simulink model "crop_simulation"  (R2021a)
settings: Solver=ode23tb  StartTime=0.0  StopTime=4  RelTol=1e-2
values from neighbouring files (symbols this model uses):
  parameters = LoadParameters()    [OnlyPlots.m]    (also in run_crop_simulation.m; run_several_crop_simulation.m)
undefined symbols (not defined in the file or in its folder): climate_GH3, MM_vec, nearst_p, p, PowerArtificial, Tr, Tref, Ts, x0_SOFC
libraries: HORTISIM x14, pid_lib x4
(part 3 of 3)

== system crop_simulation/Control Systems/Heater/SOFC cascada/Reformer + SOFC/Reformer  - SOFC System/SOFC /Nernst’s Eq  ==
  note: Hemos fijado la dimension de salida de este bloque
  note: 'H2' , 'O2' , 'H2O' , 'N2' , 'CO' , 'CH4' , 'CO2' , 'Diesel' ,'Ar','Csoot'
  Xa : Inport
  I : Inport  Port=2
  T : Inport  Port=3
  ratio a/c : Inport  Port=4
  Constant5 : Constant  Value=nearst_p.mu_out
  Gain : Gain  Gain=nearst_p.std_out
  MATLAB Function1 : MATLAB Function  TreatAsAtomicUnit=on
  Scope1 : Scope
  Subsystem : Subsystem
  Subsystem1 : Subsystem  Variant=on  VariantControlMode=label  VariantControl=Choice  LabelModeActiveChoice=Choice_1
  Sum : Sum  Inputs=|++
  V : Outport  PortDimensions=1
  wires:
  T/1 -> Subsystem/2(T)
  Xa/1 -> Subsystem/3(la)
  ratio a/c/1 -> Subsystem/1(ratio a/c)
  Gain/1 -> Sum/1
  Constant5/1 -> Sum/2
  Sum/1 -> Scope1/1, MATLAB Function1/1(params)
  MATLAB Function1/1(V) -> V/1
  I/1 -> MATLAB Function1/2(I)
  Subsystem/1(Out7) -> Subsystem1/1(In1)
  Subsystem1/1(Out1) -> Gain/1

== system crop_simulation/Control Systems/Heater/SOFC cascada/Reformer + SOFC/Reformer  - SOFC System/SOFC /Subsystem ==
  Air[mol/s] : Inport
  Molar Fractions (H2,O2,H2O,N2,CO,CH4,CO2) [mol/(Air-mol)] : Constant  Value=[0 0.2095 0 0.7808 0 0 0 0 0 0]
  Product : Product
  Cathode [mol/s] : Outport
  wires:
  Air[mol/s]/1 -> Product/1  "Air [mol/s]"
  Product/1 -> Cathode [mol/s]/1  "Cathode [mol/s]"
  Molar Fractions (H2,O2,H2O,N2,CO,CH4,CO2) [mol/(Air-mol)]/1 -> Product/2

== system crop_simulation/Control Systems/Heater/SOFC/Reformer  - SOFC System/Reformer /Subsystem/Subsystem/Subsystem ==
  In1 : Inport
  Equilibrium : MATLABFcn  MATLABFcn=forward_reformer_net  OutputDimensions=8  OutputSignalType=real  Output1D=off
  Out1 : Outport
  wires:
  In1/1 -> Equilibrium/1
  Equilibrium/1 -> Out1/1

== system crop_simulation/Control Systems/Heater/SOFC/Reformer  - SOFC System/Reformer /Subsystem/Subsystem/Subsystem1 ==
  In1 : Inport
  MATLAB Function : MATLAB Function  TreatAsAtomicUnit=on
  Out1 : Outport

== system crop_simulation/Control Systems/Heater/SOFC/Reformer  - SOFC System/Reformer /Subsystem/Subsystem1/Subsystem ==
  In1 : Inport
  MATLAB Function : MATLAB Function  TreatAsAtomicUnit=on
  Out1 : Outport

== system crop_simulation/Control Systems/Heater/SOFC/Reformer  - SOFC System/Reformer /Subsystem/Subsystem1/Subsystem1 ==
  In1 : Inport
  Inlet Composition : MATLABFcn  MATLABFcn=inlet_reformer_net  OutputDimensions=6  OutputSignalType=real  Output1D=off
  Out1 : Outport
  wires:
  In1/1 -> Inlet Composition/1
  Inlet Composition/1 -> Out1/1

== system crop_simulation/Control Systems/Heater/SOFC/Reformer  - SOFC System/SOFC /Nernst’s Eq /Subsystem1/Subsystem ==
  In1 : Inport
  MATLAB Function : MATLAB Function  TreatAsAtomicUnit=on
  Out1 : Outport
  wires:
  In1/1 -> MATLAB Function/1(u)
  MATLAB Function/1(y) -> Out1/1

== system crop_simulation/Control Systems/Heater/SOFC/Reformer  - SOFC System/SOFC /Nernst’s Eq /Subsystem1/Subsystem1 ==
  In1 : Inport
  Interpreted MATLAB Function : MATLABFcn  MATLABFcn=nearst_nn
  Out1 : Outport
  wires:
  In1/1 -> Interpreted MATLAB Function/1
  Interpreted MATLAB Function/1 -> Out1/1

== system crop_simulation/Control Systems/Heater/SOFC cascada/Control Operations Points/Control OP/Select Operation Point/Select Operation Point/If Action Subsystem ==
  Action Port : ActionPort
  Constant : Constant  Value=4
  Out1 : Outport
  wires:
  Constant/1 -> Out1/1

== system crop_simulation/Control Systems/Heater/SOFC cascada/Control Operations Points/Control OP/Select Operation Point/Select Operation Point/If Action Subsystem1 ==
  Action Port : ActionPort
  Constant : Constant  Value=3
  Out1 : Outport
  wires:
  Constant/1 -> Out1/1

== system crop_simulation/Control Systems/Heater/SOFC cascada/Control Operations Points/Control OP/Select Operation Point/Select Operation Point/If Action Subsystem2 ==
  Action Port : ActionPort
  Constant : Constant
  Out1 : Outport
  wires:
  Constant/1 -> Out1/1

== system crop_simulation/Control Systems/Heater/SOFC cascada/Control Operations Points/Control OP/Transformacion Flujos/If Action Subsystem/Subsystem ==
  Constant : Constant  Value=11.64
  Constant1 : Constant  Value=14.14
  Constant2 : Constant  Value=36.18
  Constant3 : Constant  Value=144
  Out Bus Element : Outport  PortName=OP  Element=Diesel [ml/min]
  Out Bus Element1 : Outport  PortName=OP  Element=Steam [ml/min]
  Out Bus Element2 : Outport  PortName=OP  Element=Air [NL/min]
  Out Bus Element3 : Outport  PortName=OP  Element=Air_cath [NL/min]
  wires:
  Constant1/1 -> Out Bus Element1/1
  Constant2/1 -> Out Bus Element2/1
  Constant/1 -> Out Bus Element/1
  Constant3/1 -> Out Bus Element3/1

== system crop_simulation/Control Systems/Heater/SOFC cascada/Control Operations Points/Control OP/Transformacion Flujos/If Action Subsystem1/Subsystem1 ==
  Constant : Constant  Value=7.83
  Constant1 : Constant  Value=9.51
  Constant2 : Constant  Value=24.34
  Constant3 : Constant  Value=96
  Out Bus Element : Outport  PortName=OP  Element=Diesel [ml/min]
  Out Bus Element1 : Outport  PortName=OP  Element=Steam [ml/min]
  Out Bus Element2 : Outport  PortName=OP  Element=Air [NL/min]
  Out Bus Element3 : Outport  PortName=OP  Element=Air_cath [NL/min]
  wires:
  Constant1/1 -> Out Bus Element1/1
  Constant2/1 -> Out Bus Element2/1
  Constant/1 -> Out Bus Element/1
  Constant3/1 -> Out Bus Element3/1

== system crop_simulation/Control Systems/Heater/SOFC cascada/Control Operations Points/Control OP/Transformacion Flujos/If Action Subsystem2/Subsystem2 ==
  Constant : Constant  Value=6.51
  Constant1 : Constant  Value=7.91
  Constant2 : Constant  Value=20.24
  Constant3 : Constant  Value=80
  Out Bus Element : Outport  PortName=OP  Element=Diesel [ml/min]
  Out Bus Element1 : Outport  PortName=OP  Element=Steam [ml/min]
  Out Bus Element2 : Outport  PortName=OP  Element=Air [NL/min]
  Out Bus Element3 : Outport  PortName=OP  Element=Air_cath [NL/min]
  wires:
  Constant1/1 -> Out Bus Element1/1
  Constant2/1 -> Out Bus Element2/1
  Constant/1 -> Out Bus Element/1
  Constant3/1 -> Out Bus Element3/1

== system crop_simulation/Control Systems/Heater/SOFC cascada/Control Operations Points/Control OP/Transformacion Flujos/If Action Subsystem3/Subsystem2 ==
  Constant : Constant  Value=4.41
  Constant1 : Constant  Value=5.36
  Constant2 : Constant  Value=13.72
  Constant3 : Constant  Value=55
  Out Bus Element : Outport  PortName=OP  Element=Diesel [ml/min]
  Out Bus Element1 : Outport  PortName=OP  Element=Steam [ml/min]
  Out Bus Element2 : Outport  PortName=OP  Element=Air [NL/min]
  Out Bus Element3 : Outport  PortName=OP  Element=Air_cath [NL/min]
  wires:
  Constant1/1 -> Out Bus Element1/1
  Constant2/1 -> Out Bus Element2/1
  Constant/1 -> Out Bus Element/1
  Constant3/1 -> Out Bus Element3/1

== system crop_simulation/Control Systems/Heater/SOFC cascada/Reformer + SOFC/Reformer  - SOFC System/Reformer /Subsystem/Order Data ==
  note: Target
  note: Target
  note: 'H2' , 'O2' , 'H2O' , 'N2' , 'CO' , 'CH4' , 'CO2' , 'Diesel' ,'Ar','Csoot'
  In1 : Inport
  Demux : Demux  Outputs=8
  Vector Concatenate : Concatenate  NumInputs=10
  Out1 : Outport
  wires:
  In1/1 -> Demux/1
  Demux/1 -> [Ar]
  Demux/2 -> [CH4]
  Demux/3 -> [CO]
  Demux/4 -> [CO2]
  Demux/5 -> [H2]
  Demux/6 -> [H2O]
  Demux/7 -> [N2]
  Demux/8 -> [Csoot]
  [H2] -> Vector Concatenate/1
  [H2O] -> Vector Concatenate/3
  [N2] -> Vector Concatenate/4
  [CO] -> Vector Concatenate/5
  [CH4] -> Vector Concatenate/6
  [CO2] -> Vector Concatenate/7
  [Ar] -> Vector Concatenate/9
  [Csoot] -> Vector Concatenate/10
  Vector Concatenate/1 -> Out1/1

== system crop_simulation/Control Systems/Heater/SOFC cascada/Reformer + SOFC/Reformer  - SOFC System/Reformer /Subsystem/Order Data1 ==
  note: 'H2' , 'O2' , 'H2O' , 'N2' , 'CO' , 'CH4' , 'CO2' , 'Diesel' ,'Ar','Csoot'
  In1 : Inport
  Demux : Demux  Outputs=6
  Vector Concatenate : Concatenate  NumInputs=10
  Out1 : Outport
  wires:
  In1/1 -> Demux/1
  Demux/1 -> [N2]
  Demux/2 -> [O2]
  Demux/3 -> [CO2]
  Demux/4 -> [H2O]
  Demux/5 -> [Ar]
  Demux/6 -> [Diesel]
  [H2O] -> Vector Concatenate/3
  [N2] -> Vector Concatenate/4
  [CO2] -> Vector Concatenate/7
  [Ar] -> Vector Concatenate/9
  Vector Concatenate/1 -> Out1/1
  [O2] -> Vector Concatenate/2
  [Diesel] -> Vector Concatenate/8

== system crop_simulation/Control Systems/Heater/SOFC cascada/Reformer + SOFC/Reformer  - SOFC System/Reformer /Subsystem/Subsystem ==
  In1 : Inport
  Subsystem : Subsystem  VariantControl=Choice
  Subsystem1 : Subsystem  VariantControl=Choice_1
  Out1 : Outport

== system crop_simulation/Control Systems/Heater/SOFC cascada/Reformer + SOFC/Reformer  - SOFC System/Reformer /Subsystem/Subsystem1 ==
  In1 : Inport
  Subsystem : Subsystem  VariantControl=Choice_1
  Subsystem1 : Subsystem  VariantControl=Choice
  Out1 : Outport

== system crop_simulation/Control Systems/Heater/SOFC cascada/Reformer + SOFC/Reformer  - SOFC System/Reformer /Subsystem1/Ainhoa ==
  Mass Flow : Inport
  T : Inport  Port=2
  Deactivation : Subsystem  mask{k0=parameters.Heating.Reformer.deactivation.k0, k=parameters.Heating.Reformer.deactivation.k, nd=parameters.Heating.Reformer.deactivation.nd, Kw_ast=parameters.Heating.Reformer.deactivation.Kw_ast, Ew=parameters.Heating.Reformer.deactivation.Ew}
  activity : Outport
  wires:
  Deactivation/1(Out1) -> activity/1
  Mass Flow/1 -> Deactivation/1(mf)
  T/1 -> Deactivation/2(T)

== system crop_simulation/Control Systems/Heater/SOFC cascada/Reformer + SOFC/Reformer  - SOFC System/Reformer /Subsystem1/Simple ==
  Gain : Gain  Gain=0
  Integrator : Integrator  InitialCondition=1
  seconds 2 days1 : Gain  Gain=3600*24*0.001
  activity : Outport
  wires:
  Integrator/1 -> activity/1, Gain/1
  seconds 2 days1/1 -> Integrator/1
  Gain/1 -> seconds 2 days1/1

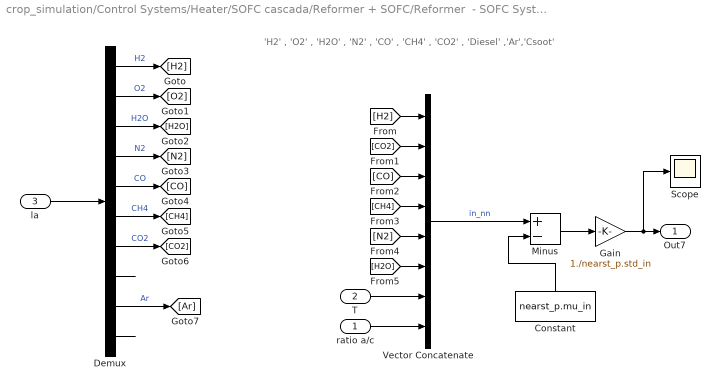
== system crop_simulation/Control Systems/Heater/SOFC cascada/Reformer + SOFC/Reformer  - SOFC System/SOFC /Nernst’s Eq /Subsystem ==
  note: 'H2' , 'O2' , 'H2O' , 'N2' , 'CO' , 'CH4' , 'CO2' , 'Diesel' ,'Ar','Csoot'
  ratio a/c : Inport
  T : Inport  Port=2
  la : Inport  Port=3
  Constant : Constant  Value=nearst_p.mu_in
  Demux : Demux  Outputs=10
  Gain : Gain  Gain=1./nearst_p.std_in
  Minus : Sum  Inputs=+-
  Scope : Scope
  Vector Concatenate : Concatenate  NumInputs=8
  Out7 : Outport
  wires:
  Demux/7 -> [CO2]  "CO2"
  la/1 -> Demux/1
  Demux/3 -> [H2O]  "H2O"
  Demux/1 -> [H2]  "H2"
  Demux/8 -> ?
  Demux/2 -> [O2]  "O2"
  Demux/10 -> ?
  Demux/9 -> [Ar]  "Ar"
  Demux/5 -> [CO]  "CO"
  Demux/4 -> [N2]  "N2"
  Demux/6 -> [CH4]  "CH4"
  ratio a/c/1 -> Vector Concatenate/8
  T/1 -> Vector Concatenate/7
  [H2] -> Vector Concatenate/1
  [CO2] -> Vector Concatenate/2
  [CO] -> Vector Concatenate/3
  [CH4] -> Vector Concatenate/4
  [N2] -> Vector Concatenate/5
  [H2O] -> Vector Concatenate/6
  Vector Concatenate/1 -> Minus/1  "in_nn"
  Constant/1 -> Minus/2
  Minus/1 -> Gain/1
  Gain/1 -> Scope/1, Out7/1

== system crop_simulation/Control Systems/Heater/SOFC cascada/Reformer + SOFC/Reformer  - SOFC System/SOFC /Nernst’s Eq /Subsystem1 ==
  In1 : Inport
  Subsystem : Subsystem  VariantControl=Choice_1
  Subsystem1 : Subsystem  VariantControl=Choice
  Out1 : Outport

== system crop_simulation/Control Systems/Heater/SOFC cascada/Reformer + SOFC/Reformer  - SOFC System/Reformer /Subsystem/Subsystem/Subsystem ==
  In1 : Inport
  Equilibrium : MATLABFcn  MATLABFcn=forward_reformer_net  OutputDimensions=8  OutputSignalType=real  Output1D=off
  Out1 : Outport
  wires:
  In1/1 -> Equilibrium/1
  Equilibrium/1 -> Out1/1

== system crop_simulation/Control Systems/Heater/SOFC cascada/Reformer + SOFC/Reformer  - SOFC System/Reformer /Subsystem/Subsystem/Subsystem1 ==
  In1 : Inport
  MATLAB Function : MATLAB Function  TreatAsAtomicUnit=on
  Out1 : Outport
  wires:
  In1/1 -> MATLAB Function/1(u)
  MATLAB Function/1(y) -> Out1/1

== system crop_simulation/Control Systems/Heater/SOFC cascada/Reformer + SOFC/Reformer  - SOFC System/Reformer /Subsystem/Subsystem1/Subsystem ==
  In1 : Inport
  MATLAB Function : MATLAB Function  TreatAsAtomicUnit=on
  Out1 : Outport
  wires:
  In1/1 -> MATLAB Function/1(u)
  MATLAB Function/1(y) -> Out1/1

== system crop_simulation/Control Systems/Heater/SOFC cascada/Reformer + SOFC/Reformer  - SOFC System/Reformer /Subsystem/Subsystem1/Subsystem1 ==
  In1 : Inport
  Inlet Composition : MATLABFcn  MATLABFcn=inlet_reformer_net  OutputDimensions=6  OutputSignalType=real  Output1D=off
  Out1 : Outport
  wires:
  In1/1 -> Inlet Composition/1
  Inlet Composition/1 -> Out1/1

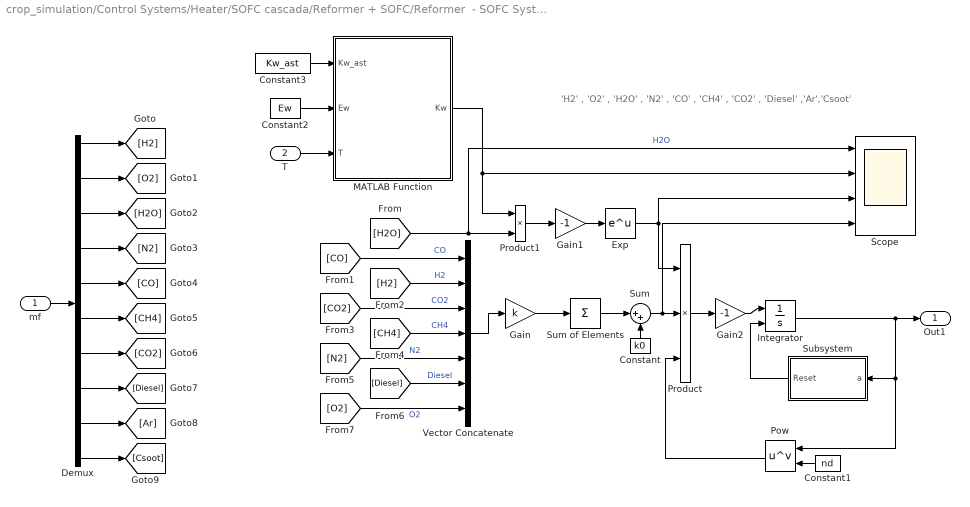
== system crop_simulation/Control Systems/Heater/SOFC cascada/Reformer + SOFC/Reformer  - SOFC System/Reformer /Subsystem1/Ainhoa/Deactivation ==
  note: 'H2' , 'O2' , 'H2O' , 'N2' , 'CO' , 'CH4' , 'CO2' , 'Diesel' ,'Ar','Csoot'
  mf : Inport
  T : Inport  Port=2
  Constant : Constant  Value=k0
  Constant1 : Constant  Value=nd
  Constant2 : Constant  Value=Ew
  Constant3 : Constant  Value=Kw_ast
  Demux : Demux  Outputs=10
  Exp : Math  SaturateOnIntegerOverflow=on
  Gain : Gain  Gain=k
  Gain1 : Gain  Gain=-1
  Gain2 : Gain  Gain=-1
  Integrator : Integrator  ExternalReset=rising  InitialCondition=1
  MATLAB Function : MATLAB Function  TreatAsAtomicUnit=on
  Pow : Math  Operator=pow  RndMeth=Zero  SaturateOnIntegerOverflow=on
  Product : Product  Inputs=3
  Product1 : Product
  Scope : Scope  NumInputPorts=4
  Subsystem : Subsystem
  Sum : Sum  Inputs=|++
  Sum of Elements : Sum  Inputs=+
  Vector Concatenate : Concatenate  NumInputs=7
  Out1 : Outport
  wires:
  Integrator/1 -> Out1/1, Subsystem/1(a), Pow/1
  mf/1 -> Demux/1
  [N2] -> Vector Concatenate/5  "N2"
  [CH4] -> Vector Concatenate/4  "CH4"
  [CO2] -> Vector Concatenate/3  "CO2"
  [H2] -> Vector Concatenate/2  "H2"
  [CO] -> Vector Concatenate/1  "CO"
  Vector Concatenate/1 -> Gain/1
  Constant/1 -> Sum/2
  Sum/1 -> Scope/4, Product/2
  [H2O] -> Scope/1, Product1/2  "H2O"
  Exp/1 -> Product/1, Scope/3
  Pow/1 -> Product/3
  Constant1/1 -> Pow/2
  Gain/1 -> Sum of Elements/1
  Sum of Elements/1 -> Sum/1
  Product/1 -> Gain2/1
  Gain2/1 -> Integrator/1
  [Diesel] -> Vector Concatenate/6  "Diesel"
  T/1 -> MATLAB Function/3(T)
  Constant2/1 -> MATLAB Function/2(Ew)
  Constant3/1 -> MATLAB Function/1(Kw_ast)
  MATLAB Function/1(Kw) -> Product1/1, Scope/2
  Product1/1 -> Gain1/1
  Gain1/1 -> Exp/1
  [O2] -> Vector Concatenate/7  "O2"
  Demux/1 -> [H2]
  Demux/2 -> [O2]
  Demux/3 -> [H2O]
  Demux/4 -> [N2]
  Demux/5 -> [CO]
  Demux/6 -> [CH4]
  Demux/7 -> [CO2]
  Demux/8 -> [Diesel]
  Demux/9 -> [Ar]
  Demux/10 -> [Csoot]
  Subsystem/1(Reset) -> Integrator/2

== system crop_simulation/Control Systems/Heater/SOFC cascada/Reformer + SOFC/Reformer  - SOFC System/SOFC /Nernst’s Eq /Subsystem1/Subsystem ==
  In1 : Inport
  MATLAB Function : MATLAB Function  TreatAsAtomicUnit=on
  Out1 : Outport
  wires:
  In1/1 -> MATLAB Function/1(u)
  MATLAB Function/1(y) -> Out1/1

== system crop_simulation/Control Systems/Heater/SOFC cascada/Reformer + SOFC/Reformer  - SOFC System/SOFC /Nernst’s Eq /Subsystem1/Subsystem1 ==
  In1 : Inport
  Interpreted MATLAB Function : MATLABFcn  MATLABFcn=nearst_nn
  Out1 : Outport
  wires:
  In1/1 -> Interpreted MATLAB Function/1
  Interpreted MATLAB Function/1 -> Out1/1

== system crop_simulation/Control Systems/Heater/SOFC cascada/Reformer + SOFC/Reformer  - SOFC System/Reformer /Subsystem1/Ainhoa/Deactivation/Subsystem ==
  a : Inport
  Constant : Constant
  Constant1 : Constant  Value=parameters.Heating.Reformer.deactivation.activity_threshold
  Delay : Delay  DelayLength=1  SampleTime=0.5/24
  Minus : Sum  Inputs=+-
  Minus1 : Sum  Inputs=+-
  Scope : Scope  NumInputPorts=2
  Sign : Signum
  Reset : Outport
  wires:
  Sign/1 -> Minus1/2
  Constant1/1 -> Minus/2
  Minus/1 -> Sign/1
  Constant/1 -> Minus1/1
  Minus1/1 -> Scope/2, Reset/1
  a/1 -> Scope/1, Delay/1
  Delay/1 -> Minus/1

== matlab function crop_simulation/Control Systems/Heater/SOFC cascada/Reformer + SOFC/Reformer  - SOFC System/Reformer /Subsystem/Subsystem1/Subsystem/MATLAB Function ==
  data: u input; y output
function y = fcn(u)

y = inlet_reformer_net(u);

== matlab function crop_simulation/Control Systems/Heater/SOFC cascada/Reformer + SOFC/Reformer  - SOFC System/SOFC /Anode/MATLAB Function ==
  data: qa_in input; ra output; I input; la output; pc_O2 input; pa input
function [ra,la] = fcn(qa_in,I,pc_O2,pa)

la = qa_in/sum(qa_in);


l_H2  = la(1);
%l_O2  = l(2);
%l_H2O = l(3);
%l_N2  = l(4);
l_CO  = la(5);
l_CH4 = la(6);
%l_CO2 = l(7);
%
alpha_H2 = l_H2;
alpha_CO  = l_CO;
alpha_CH4 = l_CH4;
%alpha_O2  = 0.5*(l_H2+l_CO+4*l_CH4);
beta_H2O  = l_H2 + 2*l_CH4;
beta_CO2  = l_CO + l_CH4;
%
F = 96485.3329; 
ne = 2*(l_H2 + l_CO + 4*l_CH4);
I = I/(F*ne);

r_H2  = -alpha_H2*I;
r_CO  = -alpha_CO*I;
r_CH4 = -alpha_CH4*I;
r_H20 = beta_H2O*I;
r_CO2 = beta_CO2*I;
%

ra = [r_H2 0 r_H20 0 r_CO r_CH4 r_CO2 0 0 0]';

sigma = 100;
eta = 5000;

theta = 0.5 + 0.5*tanh(eta*pa);
relu = theta.*(1 - exp(-pa.^2/sigma^2));

ra = ra.*relu;

%if pc_O2 <= 1e-3
%    ra  = 0*ra;
%end

== matlab function crop_simulation/Control Systems/Heater/SOFC cascada/Reformer + SOFC/Reformer  - SOFC System/SOFC /Cathode/MATLAB Function ==
  data: rc output; I input; pc_O2 input
function rc = fcn(I,pc_O2)

%l = qc_in/sum(qc_in);

% l_H2  = l(1);
% l_O2  = l(2);
% l_H2O = l(3);
% l_N2  = l(4);
% l_CO  = l(5);
% l_CH4 = l(6);
% l_CO2 = l(7);
%
% alpha_H_2 = l_H2;
% alpha_CO  = l_CO;
% alpha_CH4 = l_CH4;
% alpha_O2  = 0.5*(l_H2+l_CO+4*l_CH4);
% beta_H2O  = l_H2 + 2*l_CH4;
% beta_CO2  = l_CO + 2*l_CH4;
%
F = 96485.3329; 

% r_H2  = -alpha_H_2*I;
% r_CO  = -alpha_CO*I;
% r_CH4 = -alpha_CH4*I;
% r_H20 = beta_H2O*I;
% r_CO2 = beta_CO2*I;
%if pc_O2 <= 1e-3
%    r_O2  = 0;
%else
    r_O2  = I/(4*F);
%end

rc = [0 -r_O2 0 0 0 0 0 0 0 0]';

== matlab function crop_simulation/Control Systems/Heater/SOFC cascada/Reformer + SOFC/Reformer  - SOFC System/SOFC /Nernst’s Eq /MATLAB Function1 ==
  data: params input; V output; I input
function V = fcn(params, I)

A_esti =  params(1);
E0_esti =  params(2);
R_esti =  params(3);

m = 0.5355;
n = 0.0313;

%I = abs(I);
V = E0_esti - I.*R_esti - A_esti*log(I) - m*exp(n*I);

== matlab function crop_simulation/Control Systems/Heater/SOFC cascada/Reformer + SOFC/Reformer  - SOFC System/SOFC /Nernst’s Eq /Subsystem1/Subsystem/MATLAB Function ==
  data: u input; y output
function y = fcn(u)


y = nearst_nn(u);

== matlab function crop_simulation/Control Systems/Heater/SOFC/Reformer  - SOFC System/SOFC /Cathode/MATLAB Function ==
  data: rc output; I input; pc_O2 input
function rc = fcn(I,pc_O2)

%l = qc_in/sum(qc_in);

% l_H2  = l(1);
% l_O2  = l(2);
% l_H2O = l(3);
% l_N2  = l(4);
% l_CO  = l(5);
% l_CH4 = l(6);
% l_CO2 = l(7);
%
% alpha_H_2 = l_H2;
% alpha_CO  = l_CO;
% alpha_CH4 = l_CH4;
% alpha_O2  = 0.5*(l_H2+l_CO+4*l_CH4);
% beta_H2O  = l_H2 + 2*l_CH4;
% beta_CO2  = l_CO + 2*l_CH4;
%
F = 96485.3329; 

% r_H2  = -alpha_H_2*I;
% r_CO  = -alpha_CO*I;
% r_CH4 = -alpha_CH4*I;
% r_H20 = beta_H2O*I;
% r_CO2 = beta_CO2*I;
%if pc_O2 <= 1e-3
%    r_O2  = 0;
%else
    r_O2  = I/(4*F);
%end

rc = [0 -r_O2 0 0 0 0 0 0 0 0]';

== matlab function crop_simulation/Control Systems/Heater/SOFC cascada/Battery/Calculo de Corriente atraves de la celda de combustible/Subsystem2/MATLAB Function ==
  data: Target input; y output; FPD input; upre input
function y = fcn(Target,FPD,upre)

y = upre + 0.005*(Target  - FPD);
y = min(y,30);
y = max(y,0.1);

== matlab function crop_simulation/Control Systems/Heater/SOFC cascada/Reformer + SOFC/Reformer  - SOFC System/Reformer /Subsystem1/Ainhoa/Deactivation/MATLAB Function ==
  data: Kw_ast input; Kw output; Ew input; T input
function Kw = fcn(Kw_ast,Ew,T)

R = 8.314472;% J/(mol K) 

Kw = Kw_ast*exp(-Ew/R*(1/(T+273.15) - 1/573));

== matlab function crop_simulation/Control Systems/Heater/SOFC/Reformer  - SOFC System/SOFC /Anode/MATLAB Function ==
  data: qa_in input; ra output; I input; la output; pc_O2 input; pa input
function [ra,la] = fcn(qa_in,I,pc_O2,pa)

la = qa_in/sum(qa_in);


l_H2  = la(1);
%l_O2  = l(2);
%l_H2O = l(3);
%l_N2  = l(4);
l_CO  = la(5);
l_CH4 = la(6);
%l_CO2 = l(7);
%
alpha_H2 = l_H2;
alpha_CO  = l_CO;
alpha_CH4 = l_CH4;
%alpha_O2  = 0.5*(l_H2+l_CO+4*l_CH4);
beta_H2O  = l_H2 + 2*l_CH4;
beta_CO2  = l_CO + l_CH4;
%
F = 96485.3329; 
ne = 2*(l_H2 + l_CO + 4*l_CH4);
I = I/(F*ne);

r_H2  = -alpha_H2*I;
r_CO  = -alpha_CO*I;
r_CH4 = -alpha_CH4*I;
r_H20 = beta_H2O*I;
r_CO2 = beta_CO2*I;
%

ra = [r_H2 0 r_H20 0 r_CO r_CH4 r_CO2 0 0 0]';

sigma = 100;
eta = 5000;

theta = 0.5 + 0.5*tanh(eta*pa);
relu = theta.*(1 - exp(-pa.^2/sigma^2));

ra = ra.*relu;

%if pc_O2 <= 1e-3
%    ra  = 0*ra;
%end

== matlab function crop_simulation/Control Systems/Heater/SOFC/Subsystem2/Subsystem2/MATLAB Function ==
  data: Target input; y output; FPD input; upre input
function y = fcn(Target,FPD,upre)

y = upre + 0.005*(Target  - FPD);
y = min(y,30);
y = max(y,0.1);

== matlab function crop_simulation/Crop Control/Lighting System /Lighting System /MATLAB Function1 ==
  data: slope input; on_off output
function on_off = fcn(slope)

on_off = 0.5+0.5*sign(slope);

== matlab function crop_simulation/Control Systems/Heater/SOFC/Reformer  - SOFC System/SOFC /Nernst’s Eq /MATLAB Function1 ==
  data: params input; V output; I input
function V = fcn(params, I)

A_esti =  params(1);
E0_esti =  params(2);
R_esti =  params(3);

m = 0.5355;
n = 0.0313;

%I = abs(I);
V = E0_esti - I.*R_esti - A_esti*log(I) - m*exp(n*I);

== matlab function crop_simulation/Control Systems/Heater/SOFC/Control OP/Select Operation Point/Relay 3/MATLAB Function ==
  data: Tw input; next_state output; state input
function next_state = fcn(Tw, state)
 
%%
% Tw     = [80, 75  ,  50 , 20]
% state  = [OP1,OP2 , OP3, OP4]
%
T1_plus = 80; 

T2_plus = 60;
T2_minus = 90; 

T3_plus = 70;
T3_minus = 85;

T4_minus = 80;

next_state = state;
switch state
    case 1
        if Tw < T1_plus
            next_state = 2;
        end
    case 2
        if Tw < T2_plus 
            next_state = 3;
        elseif Tw > T2_minus
            next_state = 1;
        end
    case 3
        if Tw < T3_plus 
            next_state = 4;
        elseif Tw > T3_minus
            next_state = 2;
        end
    case 4
        if Tw > T4_minus 
            next_state = 3;
        end
end

== matlab function crop_simulation/Control Systems/Heater/SOFC/Reformer  - SOFC System/SOFC /Nernst’s Eq /Subsystem1/Subsystem/MATLAB Function ==
  data: u input; y output
function y = fcn(u)


y = nearst_nn(u);

== matlab function crop_simulation/Control Systems/Heater/SOFC/Reformer  - SOFC System/Reformer /Subsystem/Subsystem/Subsystem1/MATLAB Function ==
  data: u input; y output
function y = fcn(u)

y = forward_reformer_net(u);

== matlab function crop_simulation/Control Systems/Heater/SOFC/Reformer  - SOFC System/Reformer /Subsystem/Subsystem1/Subsystem/MATLAB Function ==
  data: u input; y output
function y = fcn(u)

y = inlet_reformer_net(u);

== matlab function crop_simulation/Control Systems/Heater/SOFC cascada/Control Operations Points/Control OP/Select Operation Point/Relay 3/MATLAB Function ==
  data: Pre_Error input; Error input; next_state output; state input
function next_state = fcn(Pre_Error, Error, state)
 


next_state = state;

if Pre_Error < -2
    if Error > 5 
        next_state = next_state + 1;
    elseif Error < -5 
        next_state = next_state - 1;
    end
elseif Pre_Error > 2 
    if Error > 5 
        next_state = next_state + 1;
    elseif Error < -5 
        next_state = next_state - 1;
    end
    
end


next_state = max(next_state,1);
next_state = min(next_state,4);

== matlab function crop_simulation/Control Systems/Heater/SOFC cascada/Reformer + SOFC/Reformer  - SOFC System/Reformer /Subsystem/Subsystem/Subsystem1/MATLAB Function ==
  data: u input; y output
function y = fcn(u)

y = forward_reformer_net(u);
